simulink subsystem "validation"  (R2020b)
settings: Solver=VariableStepAuto  StartTime=0.0  StopTime=10.0  RelTol=1e-3
settings Model: Creator=billy  LastModifiedBy=billy

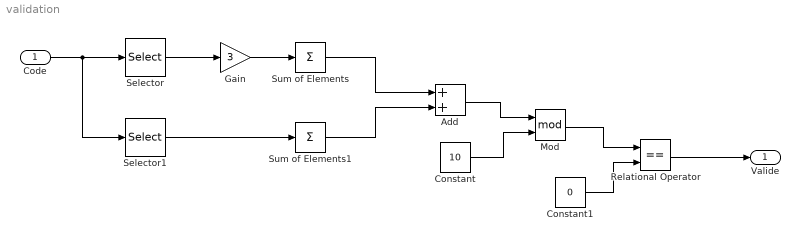
== system validation ==
  Code : Inport
  Add : Sum
  Constant : Constant  Value=10
  Constant1 : Constant  Value=0
  Gain : Gain  Gain=3
  Mod : Math  Operator=mod  OutputSignalType=real  SaturateOnIntegerOverflow=on
  Relational Operator : RelationalOperator  Operator===  OutDataTypeStr=boolean  RndMeth=Simplest
  Selector : Selector  InputPortWidth=12  IndexOptions=Index vector (dialog)  Indices=[1 3 5 7 9 11]  OutputSizes=1
  Selector1 : Selector  InputPortWidth=12  IndexOptions=Index vector (dialog)  Indices=[2 4 6 8 10 12]  OutputSizes=1
  Sum of Elements : Sum  Inputs=+
  Sum of Elements1 : Sum  Inputs=+
  Valide : Outport  OutDataTypeStr=boolean
  wires:
  Code/1 -> Selector1/1, Selector/1
  Selector/1 -> Gain/1
  Gain/1 -> Sum of Elements/1
  Selector1/1 -> Sum of Elements1/1
  Sum of Elements/1 -> Add/1
  Sum of Elements1/1 -> Add/2
  Add/1 -> Mod/1
  Constant/1 -> Mod/2
  Mod/1 -> Relational Operator/1
  Constant1/1 -> Relational Operator/2
  Relational Operator/1 -> Valide/1
